simulink model "elen110lab6"  (R2026a)
settings: Solver=VariableStepAuto  StopTime=20.0

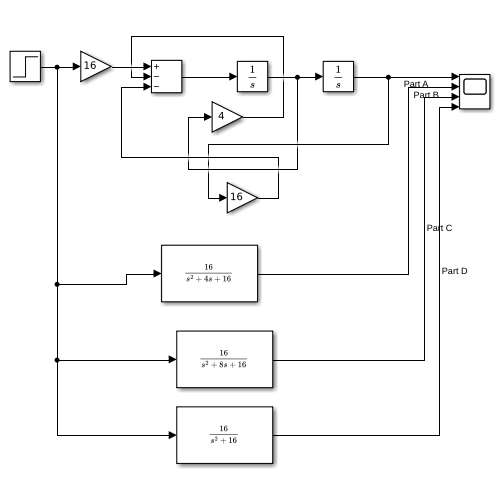
[thumbnail: Simulink's stored preview of the top-level diagram]
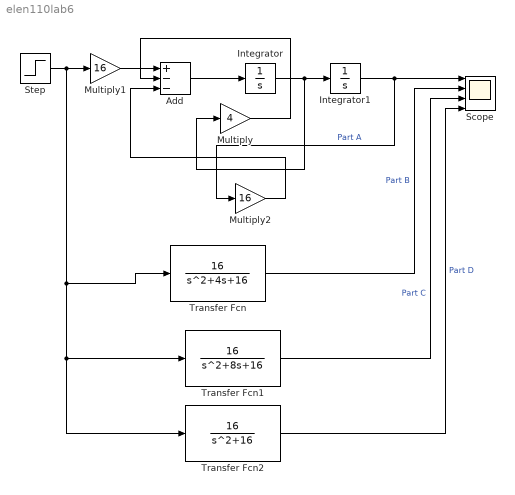
== system elen110lab6 ==
  Add : Sum  Inputs=+--
  Integrator : Integrator
  Integrator1 : Integrator
  Multiply : Gain  Gain=4
  Multiply1 : Gain  Gain=16
  Multiply2 : Gain  Gain=16
  Scope : Scope  NumInputPorts=4
      settings: ActiveDisplayYMinimum=-0.24997865307815029  ActiveDisplayYMaximum=2.2498078777033532
  Step : Step  Time=5  SampleTime=0
  Transfer Fcn : TransferFcn  Numerator=[16]  Denominator=[1 4 16]
  Transfer Fcn1 : TransferFcn  Numerator=[16]  Denominator=[1 8 16]
  Transfer Fcn2 : TransferFcn  Numerator=[16]  Denominator=[1 0 16]
  wires:
  Add/1 -> Integrator/1
  Integrator/1 -> Multiply/1, Integrator1/1
  Integrator1/1 -> Multiply2/1, Scope/1  "Part A"
  Multiply/1 -> Add/2
  Step/1 -> Transfer Fcn2/1, Transfer Fcn1/1, Transfer Fcn/1, Multiply1/1
  Multiply1/1 -> Add/1
  Multiply2/1 -> Add/3
  Transfer Fcn/1 -> Scope/2  "Part B"
  Transfer Fcn1/1 -> Scope/3  "Part C"
  Transfer Fcn2/1 -> Scope/4  "Part D"
